simulink model "lqictrl17"  (R2017a)
settings: Solver=ode1  StartTime=0.0  StopTime=20  FixedStep=0.002  RelTol=1e-3  EnableMultiTasking=on
values from neighbouring files (symbols this model uses):
  A = [0 0 1 0 ... (first row only)    [lqrintctrl.m]
  B = [0;0;51.5346;-49.3846]    [lqrintctrl.m]
  C = [1 0 0 0;0 1 0 0]    [lqrintctrl.m]
  D = [0;0]    [lqrintctrl.m]
  wcf_1 = 2 * pi * 50    (= 314.159265359)    [lqrintctrl.m]
  wcf_2 = 2 * pi * 10    (= 62.8318530718)    [lqrintctrl.m]
libraries: simulink_extras x2, simulink x1
settings Model: ExtModeTrigDuration=5000  Creator=MLevis  LastModifiedBy=frank
settings SolverCC: PositivePriorityOrder=on
settings DataIOCC: LimitDataPoints=on  SaveFormat=Array  SignalLoggingSaveFormat=ModelDataLogs
settings OptimizationCC: ExpressionDepthLimit=2147483647  InitFltsAndDblsToZero=on  LifeSpan=inf
settings DebuggingCC: SaveWithParameterizedLinksMsg=none  UnderspecifiedInitializationDetection=Classic  MergeDetectMultiDrivingBlocksExec=none  SolverPrmCheckMsg=warning  FcnCallInpInsideContextMsg=warning  StateNameClashWarn=warning  SFUnexpectedBacktrackingDiag=warning  SFNoUnconditionalDefaultTransitionDiag=warning  SFExecutionAtInitializationDiag=none
settings HardwareCC: ProdBitPerPointer=32  ProdBitPerSizeT=32  ProdBitPerPtrDiffT=32  ProdLargestAtomicFloat=None  ProdIntDivRoundTo=Undefined  ProdEndianess=Unspecified  ProdWordSize=32  ProdHWDeviceType=32-bit Generic
settings ModelReferenceCC: PropagateSignalLabelsOutOfModel=off
settings SFSimCC: SimUseLocalCustomCode=on
settings RTWCC: Description=QUARC Win32 Target  SystemTargetFile=quarc_windows.tlc  TemplateMakefile=quarc_default_tmf  RTWUseLocalCustomCode=on
settings STFCustomTargetCC: TargetFcnLib=ansi_tfl_tmw.mat  TargetPreCompLibLocation=C:\DOCUME~1\ALLUSE~1\APPLIC~1\QUARC\lib\2007a\windows\release  CPPClassGenCompliant=on  SystemTargetFile=quarc_windows.tlc
settings GRTTargetCC: TargetFcnLib=ansi_tfl_tmw.mat  TargetPreCompLibLocation=C:\DOCUME~1\ALLUSE~1\APPLIC~1\QUARC\lib\2007a\windows\release  TargetLangStandard=C89/C90 (ANSI)  ParMdlRefBuildCompliant=off  CompOptLevelCompliant=off  ConcurrentExecutionCompliant=off  CombineOutputUpdateFcns=off  MatFileLogging=off  GRTInterface=on  UseToolchainInfoCompliant=off  ExtMode=on  ExtModeMexFile=quarc_comm
settings ConfigComp: CovMetricSettings=dw  CovHtmlReporting=on  CovSaveCumulativeToWorkspaceVar=on  CovSaveSingleToWorkspaceVar=on

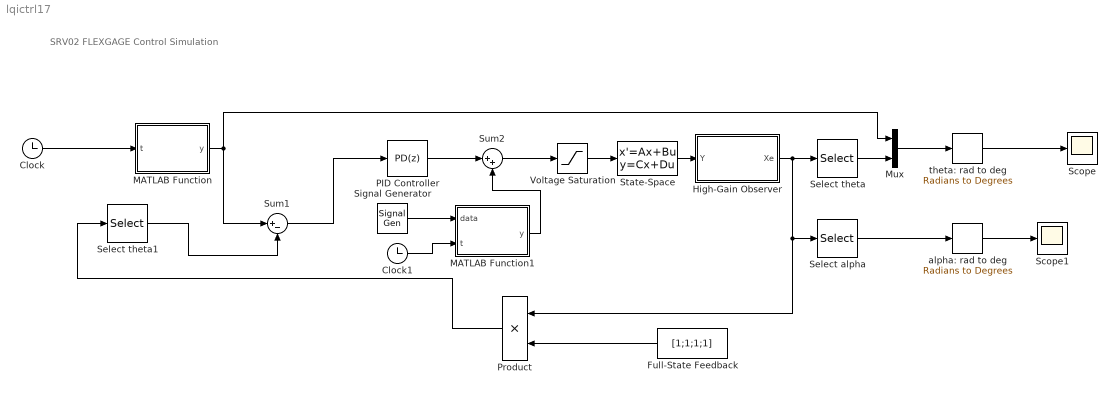
== system lqictrl17 ==
  note: SRV02 FLEXGAGE Control Simulation
  Clock : Clock
  Clock1 : Clock
  Full-State Feedback : Constant  Value=[1;1;1;1]
  High-Gain Observer : Subsystem
  MATLAB Function : MATLAB Function  TreatAsAtomicUnit=on
  MATLAB Function1 : MATLAB Function  TreatAsAtomicUnit=on
  Mux : Mux  Inputs=2
  PID Controller : simulink/Continuous/PID Controller  Controller=PD  Form=Parallel  TimeDomain=Discrete-time  SampleTime=-1  IntegratorMethod=Forward Euler  FilterMethod=Forward Euler  ControllerParametersSource=internal  P=1.01567098102538  I=3.39497664602203e-06  D=0.80402647429883  UseFilter=on  N=37.3703754292565  InitialConditionSource=internal  InitialConditionForIntegrator=0  InitialConditionForFilter=0  DifferentiatorICPrevScaledInput=0  ExternalReset=none  TrackingMode=off  Kt=1  LimitOutput=off  UpperSaturationLimit=inf  LowerSaturationLimit=-inf  LinearizeAsGain=on  AntiWindupMode=none  Kb=1  POutMin=[]  POutMax=[]  IOutMin=[]  IOutMax=[]  DOutMin=[]  DOutMax=[]  NOutMin=[]  NOutMax=[]  SumOutMin=[]  SumOutMax=[]  SaturationOutMin=[]  SaturationOutMax=[]  PParamMin=[]  PParamMax=[]  IParamMin=[]  IParamMax=[]  DParamMin=[]  DParamMax=[]  NParamMin=[]  NParamMax=[]  KbParamMin=[]  KbParamMax=[]  KtParamMin=[]  KtParamMax=[]  KbOutMin=[]  KbOutMax=[]  KtOutMin=[]  KtOutMax=[]  IntegratorOutMin=[]  IntegratorOutMax=[]  FilterOutMin=[]  FilterOutMax=[]  SumI1OutMin=[]  SumI1OutMax=[]  SumI2OutMin=[]  SumI2OutMax=[]  SumI3OutMin=[]  SumI3OutMax=[]  SumDOutMin=[]  SumDOutMax=[]  DifferentiatorOutMin=[]  DifferentiatorOutMax=[]  IntegratorContinuousStateAttributes=''  IntegratorStateMustResolveToSignalObject=off  IntegratorRTWStateStorageClass=Auto  FilterContinuousStateAttributes=''  FilterStateMustResolveToSignalObject=off  FilterRTWStateStorageClass=Auto
  Product : Product  RndMeth=Zero
  Scope : Scope
  Scope1 : Scope
  Select alpha : Selector  InputPortWidth=4  IndexOptions=Index vector (dialog)  Indices=[2]  OutputSizes=1
  Select theta : Selector  InputPortWidth=4  IndexOptions=Index vector (dialog)  Indices=[1]  OutputSizes=1
  Select theta1 : Selector  InputPortWidth=4  IndexOptions=Index vector (dialog)  Indices=[1]  OutputSizes=1
  Signal Generator : SignalGenerator  WaveForm=square  Amplitude=0.1  Units=rad/sec
  State-Space : StateSpace  A=A  B=B  C=C  D=D  X0=[0,0,0,0]
  Sum1 : Sum  Inputs=|+-
  Sum2 : Sum  Inputs=|++
  Voltage Saturation : Saturate  UpperLimit=10  LowerLimit=-10
  alpha: rad to deg : simulink_extras/Transformations/Radians to Degrees
  theta: rad to deg : simulink_extras/Transformations/Radians to Degrees
  wires:
  Mux/1 -> theta: rad to deg/1
  Select theta/1 -> Mux/2
  Select alpha/1 -> alpha: rad to deg/1
  Full-State Feedback/1 -> Product/2
  Product/1 -> Select theta1/1
  State-Space/1 -> High-Gain Observer/1(Y)
  High-Gain Observer/1(Xe) -> Select theta/1, Product/1, Select alpha/1
  Voltage Saturation/1 -> State-Space/1
  Clock/1 -> MATLAB Function/1(t)
  MATLAB Function/1(y) -> Mux/1, Sum1/1
  theta: rad to deg/1 -> Scope/1
  alpha: rad to deg/1 -> Scope1/1
  Select theta1/1 -> Sum1/2
  Sum1/1 -> PID Controller/1
  PID Controller/1 -> Sum2/1
  Sum2/1 -> Voltage Saturation/1
  MATLAB Function1/1(y) -> Sum2/2
  Signal Generator/1 -> MATLAB Function1/1(data)
  Clock1/1 -> MATLAB Function1/2(t)

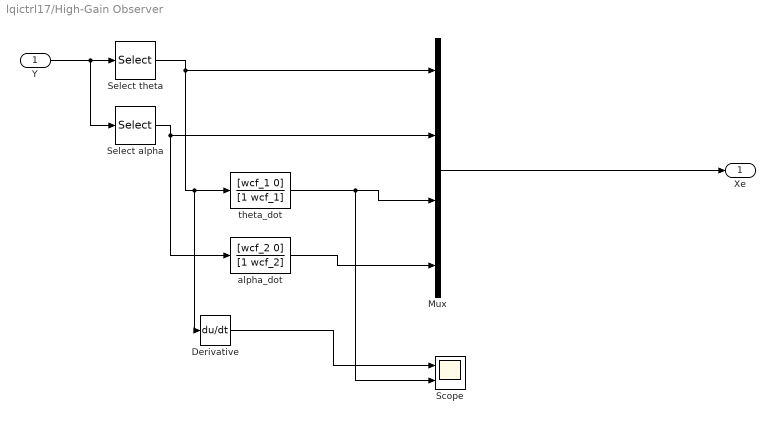
== system lqictrl17/High-Gain Observer ==
  Y : Inport
  Derivative : Derivative
  Mux : Mux
  Scope : Scope  NumInputPorts=2
  Select alpha : Selector  InputPortWidth=2  IndexOptions=Index vector (dialog)  Indices=2  OutputSizes=1
  Select theta : Selector  InputPortWidth=2  IndexOptions=Index vector (dialog)  Indices=1  OutputSizes=1
  alpha_dot : TransferFcn  Numerator=[wcf_2 0]  Denominator=[1 wcf_2]
  theta_dot : TransferFcn  Numerator=[wcf_1 0]  Denominator=[1 wcf_1]
  Xe : Outport
  wires:
  theta_dot/1 -> Scope/2, Mux/3
  alpha_dot/1 -> Mux/4
  Select alpha/1 -> alpha_dot/1, Mux/2
  Mux/1 -> Xe/1
  Y/1 -> Select alpha/1, Select theta/1
  Select theta/1 -> Derivative/1, theta_dot/1, Mux/1
  Derivative/1 -> Scope/1

== matlab function lqictrl17/MATLAB Function1 ==
  data: data input; t input; y output
function y = fcn( data,t)
if t>8 && t<10
    y=data;
else
    y=0;
end

== matlab function lqictrl17/MATLAB Function ==
  data: t input; y output
function y = fcn(t)
if t<2
    y=0;
elseif (t>=2 && t<=6)
y=-5/4096*(t-2)^7 + 35/2048*(t-2)^6 - 21/256*(t-2)^5 + 35/256*(t-2)^4;
else
   y=1
end
